simulink model "A43333_Parte2Seccion1_2y3"  (R2021a)
settings: Solver=FixedStepAuto  StartTime=0.0  StopTime=15.0  FixedStep=1e-4  RelTol=1e-3
values from neighbouring files (symbols this model uses):
  Kc = 3    [A43333_SimulacionParte2todaslasSecciones.m]
  Ve = 0    [A43333_SimulacionParte2todaslasSecciones.m]
  Vef = 1    [A43333_SimulacionParte2todaslasSecciones.m]
settings Model: Creator=Royer  LastModifiedBy=Royer

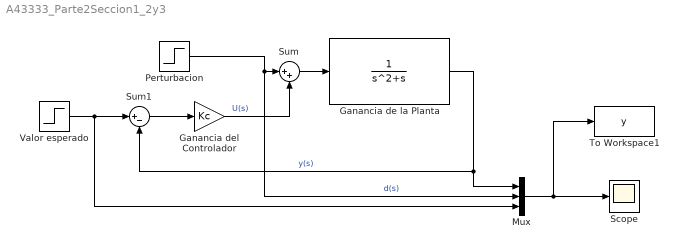
== system A43333_Parte2Seccion1_2y3 ==
  Ganancia de la Planta : TransferFcn  Denominator=[1 1 0]
  Ganancia del Controlador : Gain  Gain=Kc
  Mux : Mux  Inputs=3
  Perturbacion : Step  Time=0  After=0  SampleTime=1  VectorParams1D=off
  Scope : Scope
  Sum : Sum  Inputs=|++
  Sum1 : Sum  Inputs=|+-
  To Workspace1 : ToWorkspace  VariableName=y  SaveFormat=Timeseries  SampleTime=-1
  Valor esperado : Step  Time=0  Before=Ve  After=Vef  SampleTime=0  VectorParams1D=off
  wires:
  Ganancia del Controlador/1 -> Sum/2  "U(s)"
  Sum1/1 -> Ganancia del Controlador/1
  Sum/1 -> Ganancia de la Planta/1
  Ganancia de la Planta/1 -> Mux/1, Sum1/2  "y(s)"
  Valor esperado/1 -> Mux/3, Sum1/1
  Perturbacion/1 -> Mux/2, Sum/1  "d(s)"
  Mux/1 -> To Workspace1/1, Scope/1
